simulink model "DifferenceRCequation1"  (R2017a)
settings: Solver=VariableStepAuto  StartTime=0.0  StopTime=10.0  RelTol=1e-3
settings Model: Creator=Administrator  LastModifiedBy=Administrator

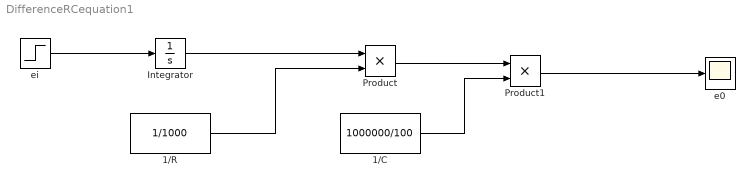
== system DifferenceRCequation1 ==
  1/C : Constant  Value=1000000/100
  1/R : Constant  Value=1/1000
  Integrator : Integrator
  Product : Product
  Product1 : Product
  e0 : Scope
  ei : Step  SampleTime=0
  wires:
  ei/1 -> Integrator/1
  Product/1 -> Product1/1
  Product1/1 -> e0/1
  Integrator/1 -> Product/1
  1/R/1 -> Product/2
  1/C/1 -> Product1/2
